simulink model "chap05"  (R2021a)
settings: Solver=FixedStepDiscrete  StartTime=0.0  StopTime=inf  FixedStep=0.001  RelTol=1e-3
undefined symbols (not defined in the file): DiscIntNeverNeededParam, Header, Pose, X, Y, Z
libraries: robotlib x31
(part 1 of 9)
settings Model: Creator=chen  LastModifiedBy=chen
settings OptimizationCC: EnhancedBackFolding=on  PassReuseOutputArgsAs=Individual arguments  ZeroExternalMemoryAtStartup=off  ZeroInternalMemoryAtStartup=off  MaxStackSize=64  OptimizeBlockOrder=speed  DifferentSizesBufferReuse=on  OptimizationCustomize=off  EfficientTunableParamExpr=on
settings DebuggingCC: ParameterTunabilityLossMsg=error
settings HardwareCC: ProdBitPerPointer=32  ProdBitPerSizeT=32  ProdBitPerPtrDiffT=32  ProdLargestAtomicFloat=None  ProdIntDivRoundTo=Undefined  ProdEndianess=Unspecified  ProdWordSize=32  ProdHWDeviceType=Generic->Unspecified (assume 32-bit Generic)
settings SFSimCC: MATLABDynamicMemAlloc=off
settings RTWCC: SystemTargetFile=ert.tlc  HardwareBoard=Robot Operating System (ROS)  TLCOptions="-aInlineSetEventsForThisBaseRateFcn=TLC_FALSE -aSuppressMultiTaskScheduler=TLC_FALSE  -aRateBasedStepFcn=0"  TemplateMakefile=ert_default_tmf  GenerateReport=on  Toolchain=Catkin  LaunchReport=on  TargetLang=C++
settings CodeAppCC: ForceParamTrailComments=on  IgnoreCustomStorageClasses=off  OperatorAnnotations=on  SimulinkDataObjDesc=on  SFDataObjDesc=on  InsertBlockDesc=on
settings ERTTargetCC: SupportContinuousTime=on

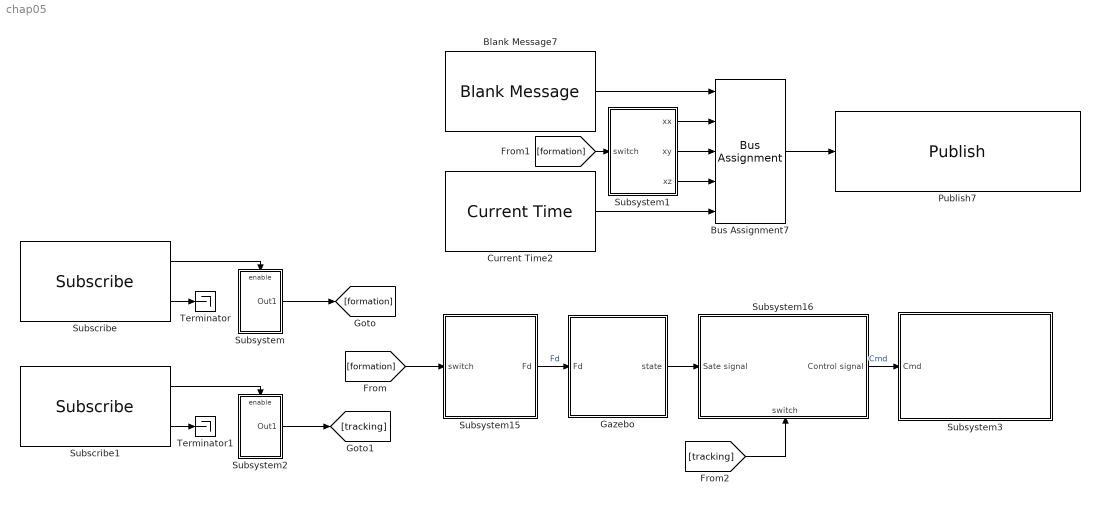
== system chap05 ==
  Blank Message7 : robotlib/Blank Message  messageClass=Message  entityType=geometry_msgs/PoseStamped  messageType=geometry_msgs/PoseStamped  SampleTime=-1  legacyBusStruct=off
  Bus Assignment7 : BusAssignment  AssignedSignals=Pose.Position.X,Pose.Position.Y,Pose.Position.Z,Header.Stamp.Sec
  Current Time2 : robotlib/Current Time  OutputFormat=double  SampleTime=-1  ModelName=chap05
      settings: SourceProductBaseCode=RR
  Gazebo : Subsystem
  Publish7 : robotlib/Publish  topicSource=Specify your own  topic=/uav0/mavros/setpoint_position/local  messageType=geometry_msgs/PoseStamped  legacyBusStruct=off  messageQueueLength=1
  Subscribe : robotlib/Subscribe  topicSource=Specify your own  topic=/start_formation  messageType=std_msgs/Empty  SampleTime=-1  legacyBusStruct=off  messageQueueLength=1
  Subscribe1 : robotlib/Subscribe  topicSource=Specify your own  topic=/start_tracking  messageType=std_msgs/Empty  SampleTime=-1  legacyBusStruct=off  messageQueueLength=1
  Subsystem : Subsystem
  Subsystem1 : Subsystem
  Subsystem15 : Subsystem
  Subsystem16 : Subsystem
      settings: PortSchema="{\"entries\":[{\"content\":{\"sides\":[{\"content\":{\"connectorIds\":[\"In1\"]},\"type\":\"ConnectorPlacement.EquallySpacedRectSide\",\"uuid\":\"50b1559e-7173-4ba8-93e6-314f6d9df527\"},{\"content\":{\"connectorIds\":[\"Out1\"],\"side\":\"RIGHT\"},\"type\":\"ConnectorPlacement.EquallySpacedRectSide\",\"uuid\":\"be527bac-0bcc-4faf-a185-0382edae0189\"},{\"content\":{\"connectorIds\":[],\"side\":\"TOP\"},\"type\":\"ConnectorPlacement.EquallySpacedRectSide\",\"uuid\":\"4c8ef68d-7cf5-4d15-9758-89dbc1169805\"},{\"content\":{\"connectorIds\":[\"In2\"],\"side\":\"BOTTOM\"},\"type\":\"ConnectorPlacement.EquallySpacedRectSide\",\"uuid\":\"887cfce8-f49d-4e35-b980-24c2ad245753\"}]},\"type\":\"ConnectorPlacement.EquallySpacedConnector\",\"uuid\":\"3c2ee67b-c3c9-431a-8107-6d5cd22b236e\"}],\"packageUris\":[\"http://schema.mathworks.com/mf0/Connector/R2020b\"],\"version\":\"1.0\"}"
  Subsystem2 : Subsystem
  Subsystem3 : Subsystem
  Terminator : Terminator
  Terminator1 : Terminator
  wires:
  [formation] -> Subsystem1/1(switch)
  Bus Assignment7/1 -> Publish7/1
  Current Time2/1 -> Bus Assignment7/5
  Blank Message7/1 -> Bus Assignment7/1
  Subsystem16/1(Control signal) -> Subsystem3/1(Cmd)  "Cmd"
  Subsystem1/1(xx) -> Bus Assignment7/2
  Subsystem1/2(xy) -> Bus Assignment7/3
  Subsystem1/3(xz) -> Bus Assignment7/4
  [tracking] -> Subsystem16/2(switch)
  Subscribe/1 -> Subsystem/Enable
  Subscribe/2 -> Terminator/1
  Subscribe1/1 -> Subsystem2/Enable
  Subscribe1/2 -> Terminator1/1
  Subsystem/1(Out1) -> [formation]
  Subsystem2/1(Out1) -> [tracking]
  [formation] -> Subsystem15/1(switch)
  Gazebo/1(state) -> Subsystem16/1(Sate signal)
  Subsystem15/1(Fd) -> Gazebo/1(Fd)  "Fd"

== system chap05/Gazebo ==
  Fd : Inport
  Bus Creator{1..4,6..8} (7 alike) : BusCreator  Inputs=6
  Bus Creator5 : BusCreator  Inputs=7
  Subscribe1 : robotlib/Subscribe  topicSource=Select from ROS network  topic=/uav1/mavros/local_position/velocity_local  messageType=geometry_msgs/TwistStamped  SampleTime=-1  legacyBusStruct=off  messageQueueLength=1
  Subscribe10 : robotlib/Subscribe  topicSource=Select from ROS network  topic=/uav4/mavros/local_position/pose  messageType=geometry_msgs/PoseStamped  SampleTime=-1  legacyBusStruct=off  messageQueueLength=1
  Subscribe11 : robotlib/Subscribe  topicSource=Select from ROS network  topic=/uav5/mavros/local_position/pose  messageType=geometry_msgs/PoseStamped  SampleTime=-1  legacyBusStruct=off  messageQueueLength=1
  Subscribe12 : robotlib/Subscribe  topicSource=Select from ROS network  topic=/uav5/mavros/local_position/velocity_local  messageType=geometry_msgs/TwistStamped  SampleTime=-1  legacyBusStruct=off  messageQueueLength=1
  Subscribe13 : robotlib/Subscribe  topicSource=Select from ROS network  topic=/uav6/mavros/local_position/pose  messageType=geometry_msgs/PoseStamped  SampleTime=-1  legacyBusStruct=off  messageQueueLength=1
  Subscribe14 : robotlib/Subscribe  topicSource=Select from ROS network  topic=/uav6/mavros/local_position/velocity_local  messageType=geometry_msgs/TwistStamped  SampleTime=-1  legacyBusStruct=off  messageQueueLength=1
  Subscribe2 : robotlib/Subscribe  topicSource=Select from ROS network  topic=/uav1/mavros/local_position/pose  messageType=geometry_msgs/PoseStamped  SampleTime=-1  legacyBusStruct=off  messageQueueLength=1
  Subscribe3 : robotlib/Subscribe  topicSource=Select from ROS network  topic=/uav3/mavros/local_position/velocity_local  messageType=geometry_msgs/TwistStamped  SampleTime=-1  legacyBusStruct=off  messageQueueLength=1
  Subscribe4 : robotlib/Subscribe  topicSource=Select from ROS network  topic=/uav3/mavros/local_position/pose  messageType=geometry_msgs/PoseStamped  SampleTime=-1  legacyBusStruct=off  messageQueueLength=1
  Subscribe5 : robotlib/Subscribe  topicSource=Select from ROS network  topic=/uav2/mavros/local_position/velocity_local  messageType=geometry_msgs/TwistStamped  SampleTime=-1  legacyBusStruct=off  messageQueueLength=1
  Subscribe6 : robotlib/Subscribe  topicSource=Select from ROS network  topic=/uav2/mavros/local_position/pose  messageType=geometry_msgs/PoseStamped  SampleTime=-1  legacyBusStruct=off  messageQueueLength=1
  Subscribe7 : robotlib/Subscribe  topicSource=Select from ROS network  topic=/uav0/mavros/local_position/velocity_local  messageType=geometry_msgs/TwistStamped  SampleTime=-1  legacyBusStruct=off  messageQueueLength=1
  Subscribe8 : robotlib/Subscribe  topicSource=Select from ROS network  topic=/uav0/mavros/local_position/pose  messageType=geometry_msgs/PoseStamped  SampleTime=-1  legacyBusStruct=off  messageQueueLength=1
  Subscribe9 : robotlib/Subscribe  topicSource=Select from ROS network  topic=/uav4/mavros/local_position/velocity_local  messageType=geometry_msgs/TwistStamped  SampleTime=-1  legacyBusStruct=off  messageQueueLength=1
  Subsystem1 : Subsystem
  Subsystem2 : Subsystem
  Subsystem3 : Subsystem
  Subsystem4 : Subsystem
  Subsystem5 : Subsystem
  Subsystem6 : Subsystem
  Subsystem7 : Subsystem
  Terminator{,1..6} (7 alike) : Terminator
  state : Outport
  wires:
  Subscribe7/2 -> Subsystem1/2(In2)
  Subscribe8/2 -> Subsystem1/1(In1)
  Subscribe8/1 -> Subsystem1/Enable
  Bus Creator1/1 -> Bus Creator5/1  "node0"
  Subsystem1/6(vz) -> Bus Creator1/6  "vz"
  Subsystem1/5(vy) -> Bus Creator1/5  "vy"
  Subsystem1/1(xx) -> Bus Creator1/1  "xx"
  Subsystem1/2(xy) -> Bus Creator1/2  "xy"
  Subsystem1/4(vx) -> Bus Creator1/4  "vx"
  Subsystem1/3(xz) -> Bus Creator1/3  "xz"
  Subsystem2/3(xz) -> Bus Creator2/3  "xz"
  Subsystem2/4(vx) -> Bus Creator2/4  "vx"
  Subsystem2/2(xy) -> Bus Creator2/2  "xy"
  Subsystem2/1(xx) -> Bus Creator2/1  "xx"
  Subsystem2/5(vy) -> Bus Creator2/5  "vy"
  Subsystem2/6(vz) -> Bus Creator2/6  "vz"
  Bus Creator2/1 -> Bus Creator5/2  "node1"
  Subscribe2/1 -> Subsystem2/Enable
  Subscribe2/2 -> Subsystem2/1(In1)
  Subscribe1/2 -> Subsystem2/2(In2)
  Subscribe1/1 -> Terminator/1
  Subscribe7/1 -> Terminator1/1
  Subscribe5/1 -> Terminator3/1
  Subscribe3/1 -> Terminator2/1
  Subscribe3/2 -> Subsystem4/2(In2)
  Subscribe4/2 -> Subsystem4/1(In1)
  Subscribe4/1 -> Subsystem4/Enable
  Bus Creator4/1 -> Bus Creator5/4  "node3"
  Subsystem4/6(vz) -> Bus Creator4/6  "vz"
  Subsystem4/5(vy) -> Bus Creator4/5  "vy"
  Subsystem4/1(xx) -> Bus Creator4/1  "xx"
  Subsystem4/2(xy) -> Bus Creator4/2  "xy"
  Subsystem4/4(vx) -> Bus Creator4/4  "vx"
  Subsystem4/3(xz) -> Bus Creator4/3  "xz"
  Subsystem3/3(xz) -> Bus Creator3/3  "xz"
  Subsystem3/4(vx) -> Bus Creator3/4  "vx"
  Subsystem3/2(xy) -> Bus Creator3/2  "xy"
  Subsystem3/1(xx) -> Bus Creator3/1  "xx"
  Subsystem3/5(vy) -> Bus Creator3/5  "vy"
  Subsystem3/6(vz) -> Bus Creator3/6  "vz"
  Bus Creator3/1 -> Bus Creator5/3  "node2"
  Subscribe6/1 -> Subsystem3/Enable
  Subscribe6/2 -> Subsystem3/1(In1)
  Subscribe5/2 -> Subsystem3/2(In2)
  Bus Creator5/1 -> state/1
  Subsystem5/3(xz) -> Bus Creator6/3  "xz"
  Subsystem5/4(vx) -> Bus Creator6/4  "vx"
  Subsystem5/2(xy) -> Bus Creator6/2  "xy"
  Subsystem5/1(xx) -> Bus Creator6/1  "xx"
  Subsystem5/5(vy) -> Bus Creator6/5  "vy"
  Subsystem5/6(vz) -> Bus Creator6/6  "vz"
  Bus Creator6/1 -> Bus Creator5/5  "node4"
  Subscribe10/1 -> Subsystem5/Enable
  Subscribe10/2 -> Subsystem5/1(In1)
  Subscribe9/2 -> Subsystem5/2(In2)
  Subscribe9/1 -> Terminator4/1
  Subscribe12/1 -> Terminator5/1
  Subscribe12/2 -> Subsystem6/2(In2)
  Subscribe11/2 -> Subsystem6/1(In1)
  Subscribe11/1 -> Subsystem6/Enable
  Bus Creator7/1 -> Bus Creator5/6  "node5"
  Subsystem6/6(vz) -> Bus Creator7/6  "vz"
  Subsystem6/5(vy) -> Bus Creator7/5  "vy"
  Subsystem6/1(xx) -> Bus Creator7/1  "xx"
  Subsystem6/2(xy) -> Bus Creator7/2  "xy"
  Subsystem6/4(vx) -> Bus Creator7/4  "vx"
  Subsystem6/3(xz) -> Bus Creator7/3  "xz"
  Subsystem7/3(xz) -> Bus Creator8/3  "xz"
  Subsystem7/4(vx) -> Bus Creator8/4  "vx"
  Subsystem7/2(xy) -> Bus Creator8/2  "xy"
  Subsystem7/1(xx) -> Bus Creator8/1  "xx"
  Subsystem7/5(vy) -> Bus Creator8/5  "vy"
  Subsystem7/6(vz) -> Bus Creator8/6  "vz"
  Bus Creator8/1 -> Bus Creator5/7  "node6"
  Subscribe13/1 -> Subsystem7/Enable
  Subscribe13/2 -> Subsystem7/1(In1)
  Subscribe14/2 -> Subsystem7/2(In2)
  Subscribe14/1 -> Terminator6/1
  Fd/1 -> Subsystem2/3(Fd), Subsystem4/3(Fd), Subsystem7/3(Fd), Subsystem6/3(Fd), Subsystem5/3(Fd), Subsystem3/3(Fd)

== system chap05/Subsystem ==
  Enable : EnablePort
  Constant3 : Constant
  Out1 : Outport  InitialOutput=0
  wires:
  Constant3/1 -> Out1/1

== system chap05/Subsystem1 ==
  switch : Inport
  Add{1..4} (4 alike) : Sum
  Constant : Constant  Value=2.5
  Constant1 : Constant  Value=pi
  Constant3 : Constant  Value=0.214
  Constant4 : Constant  Value=0.35
  Constant5 : Constant  Value=0
  Constant6 : Constant  Value=0.214
  Constant8 : Constant  Value=0.5*pi
  Product{,1..3,5} (5 alike) : Product
  Subsystem : Subsystem
      settings: PortSchema="{\"entries\":[{\"content\":{\"sides\":[{\"content\":{\"connectorIds\":[\"In1\"]},\"type\":\"ConnectorPlacement.EquallySpacedRectSide\",\"uuid\":\"50b1559e-7173-4ba8-93e6-314f6d9df527\"},{\"content\":{\"connectorIds\":[\"Out1\"],\"side\":\"RIGHT\"},\"type\":\"ConnectorPlacement.EquallySpacedRectSide\",\"uuid\":\"be527bac-0bcc-4faf-a185-0382edae0189\"},{\"content\":{\"connectorIds\":[\"In2\"],\"side\":\"TOP\"},\"type\":\"ConnectorPlacement.EquallySpacedRectSide\",\"uuid\":\"4c8ef68d-7cf5-4d15-9758-89dbc1169805\"}]},\"type\":\"ConnectorPlacement.EquallySpacedConnector\",\"uuid\":\"3c2ee67b-c3c9-431a-8107-6d5cd22b236e\"}],\"packageUris\":[\"http://schema.mathworks.com/mf0/Connector/R2020b\"],\"version\":\"1.0\"}"
  Subsystem1 : Subsystem
      settings: PortSchema="{\"entries\":[{\"content\":{\"sides\":[{\"content\":{\"connectorIds\":[\"In1\"]},\"type\":\"ConnectorPlacement.EquallySpacedRectSide\",\"uuid\":\"50b1559e-7173-4ba8-93e6-314f6d9df527\"},{\"content\":{\"connectorIds\":[\"Out1\"],\"side\":\"RIGHT\"},\"type\":\"ConnectorPlacement.EquallySpacedRectSide\",\"uuid\":\"be527bac-0bcc-4faf-a185-0382edae0189\"},{\"content\":{\"connectorIds\":[\"In2\"],\"side\":\"TOP\"},\"type\":\"ConnectorPlacement.EquallySpacedRectSide\",\"uuid\":\"4c8ef68d-7cf5-4d15-9758-89dbc1169805\"}]},\"type\":\"ConnectorPlacement.EquallySpacedConnector\",\"uuid\":\"3c2ee67b-c3c9-431a-8107-6d5cd22b236e\"}],\"packageUris\":[\"http://schema.mathworks.com/mf0/Connector/R2020b\"],\"version\":\"1.0\"}"
  Subsystem16 : Subsystem
  Trigonometric Function : Trigonometry  Operator=cos
  Trigonometric Function2 : Trigonometry  Operator=cos
  r1 : Constant  Value=4
  r2 : Constant  Value=1.5
  xx : Outport
  xy : Outport  Port=2
  xz : Outport  Port=3
  wires:
  Add2/1 -> Trigonometric Function2/1
  Trigonometric Function2/1 -> Product2/2
  Product2/1 -> Subsystem1/1(zt3)
  r1/1 -> Product2/1
  [time] -> Product5/2
  Product5/1 -> Add1/1
  Constant4/1 -> Product5/1
  Constant5/1 -> Add1/2
  Constant8/1 -> Add2/2
  Constant6/1 -> Product3/1
  [time] -> Product3/2
  Product3/1 -> Add2/1
  Trigonometric Function/1 -> Product/2
  r2/1 -> Product/1
  Add3/1 -> Trigonometric Function/1
  [time] -> Product1/2
  Constant3/1 -> Product1/1
  Product/1 -> Add4/1
  Constant/1 -> Add4/2
  Product1/1 -> Add3/1
  Constant1/1 -> Add3/2
  Add4/1 -> Subsystem/1(zt3)
  Subsystem16/1(time) -> [time]
  switch/1 -> [switch], Subsystem16/1(switch)
  Subsystem/1(Out1) -> xz/1
  [switch] -> Subsystem/2(switch)
  Subsystem1/1(xy) -> xy/1
  [switch] -> Subsystem1/2(switch)
  Add1/1 -> xx/1

== system chap05/Subsystem15 ==
  switch : Inport
  Subsystem : Subsystem
  Subsystem14 : Subsystem
  Subsystem16 : Subsystem
  Subsystem8 : Subsystem
  Switch : Switch  Criteria=u2 > Threshold  Threshold=10
  Switch1 : Switch  Criteria=u2 > Threshold  Threshold=20
  Fd : Outport
  wires:
  Switch/1 -> Switch1/3
  Subsystem16/1(time) -> Switch/2, Switch1/2
  switch/1 -> Subsystem16/1(switch)
  Subsystem14/1(Fd3) -> Switch1/1
  Subsystem8/1(Fd1) -> Switch/3
  Subsystem/1(Fd2) -> Switch/1
  Switch1/1 -> Fd/1

== system chap05/Subsystem16 ==
  Sate signal : Inport
  switch : Inport  Port=2
  Bus Creator : BusCreator  Inputs=6
  Bus Creator2 : BusCreator  Inputs=3
  Bus Creator3 : BusCreator  Inputs=6
  Subsystem : Subsystem
      settings: PortSchema="{\"entries\":[{\"content\":{\"sides\":[{\"content\":{\"connectorIds\":[\"In1\"]},\"type\":\"ConnectorPlacement.EquallySpacedRectSide\",\"uuid\":\"50b1559e-7173-4ba8-93e6-314f6d9df527\"},{\"content\":{\"connectorIds\":[\"Out1\"],\"side\":\"RIGHT\"},\"type\":\"ConnectorPlacement.EquallySpacedRectSide\",\"uuid\":\"be527bac-0bcc-4faf-a185-0382edae0189\"},{\"content\":{\"connectorIds\":[],\"side\":\"TOP\"},\"type\":\"ConnectorPlacement.EquallySpacedRectSide\",\"uuid\":\"4c8ef68d-7cf5-4d15-9758-89dbc1169805\"},{\"content\":{\"connectorIds\":[\"In2\"],\"side\":\"BOTTOM\"},\"type\":\"ConnectorPlacement.EquallySpacedRectSide\",\"uuid\":\"2cbbf04f-3669-4691-b0be-f4c904003730\"}]},\"type\":\"ConnectorPlacement.EquallySpacedConnector\",\"uuid\":\"3c2ee67b-c3c9-431a-8107-6d5cd22b236e\"}],\"packageUris\":[\"http://schema.mathworks.com/mf0/Connector/R2020b\"],\"version\":\"1.0\"}"
  Subsystem1 : Subsystem
      settings: PortSchema="{\"entries\":[{\"content\":{\"sides\":[{\"content\":{\"connectorIds\":[\"In1\"]},\"type\":\"ConnectorPlacement.EquallySpacedRectSide\",\"uuid\":\"50b1559e-7173-4ba8-93e6-314f6d9df527\"},{\"content\":{\"connectorIds\":[\"Out1\"],\"side\":\"RIGHT\"},\"type\":\"ConnectorPlacement.EquallySpacedRectSide\",\"uuid\":\"be527bac-0bcc-4faf-a185-0382edae0189\"},{\"content\":{\"connectorIds\":[],\"side\":\"TOP\"},\"type\":\"ConnectorPlacement.EquallySpacedRectSide\",\"uuid\":\"4c8ef68d-7cf5-4d15-9758-89dbc1169805\"},{\"content\":{\"connectorIds\":[\"In2\"],\"side\":\"BOTTOM\"},\"type\":\"ConnectorPlacement.EquallySpacedRectSide\",\"uuid\":\"62a0e2ad-d0ed-4a01-9855-22721dd4145c\"}]},\"type\":\"ConnectorPlacement.EquallySpacedConnector\",\"uuid\":\"3c2ee67b-c3c9-431a-8107-6d5cd22b236e\"}],\"packageUris\":[\"http://schema.mathworks.com/mf0/Connector/R2020b\"],\"version\":\"1.0\"}"
  Subsystem12 : Subsystem
  Subsystem14 : Subsystem
  Subsystem15 : Subsystem
  Subsystem16 : Subsystem
  Subsystem17 : Subsystem
  Subsystem2 : Subsystem
      settings: PortSchema="{\"entries\":[{\"content\":{\"sides\":[{\"content\":{\"connectorIds\":[\"In1\"]},\"type\":\"ConnectorPlacement.EquallySpacedRectSide\",\"uuid\":\"50b1559e-7173-4ba8-93e6-314f6d9df527\"},{\"content\":{\"connectorIds\":[\"Out1\"],\"side\":\"RIGHT\"},\"type\":\"ConnectorPlacement.EquallySpacedRectSide\",\"uuid\":\"be527bac-0bcc-4faf-a185-0382edae0189\"},{\"content\":{\"connectorIds\":[],\"side\":\"TOP\"},\"type\":\"ConnectorPlacement.EquallySpacedRectSide\",\"uuid\":\"4c8ef68d-7cf5-4d15-9758-89dbc1169805\"},{\"content\":{\"connectorIds\":[\"In2\"],\"side\":\"BOTTOM\"},\"type\":\"ConnectorPlacement.EquallySpacedRectSide\",\"uuid\":\"45420c28-548a-43d1-89f9-1bbe4c81c7d8\"}]},\"type\":\"ConnectorPlacement.EquallySpacedConnector\",\"uuid\":\"3c2ee67b-c3c9-431a-8107-6d5cd22b236e\"}],\"packageUris\":[\"http://schema.mathworks.com/mf0/Connector/R2020b\"],\"version\":\"1.0\"}"
  Subsystem3 : Subsystem
      settings: PortSchema="{\"entries\":[{\"content\":{\"sides\":[{\"content\":{\"connectorIds\":[\"In1\"]},\"type\":\"ConnectorPlacement.EquallySpacedRectSide\",\"uuid\":\"50b1559e-7173-4ba8-93e6-314f6d9df527\"},{\"content\":{\"connectorIds\":[\"Out1\"],\"side\":\"RIGHT\"},\"type\":\"ConnectorPlacement.EquallySpacedRectSide\",\"uuid\":\"be527bac-0bcc-4faf-a185-0382edae0189\"},{\"content\":{\"connectorIds\":[],\"side\":\"TOP\"},\"type\":\"ConnectorPlacement.EquallySpacedRectSide\",\"uuid\":\"4c8ef68d-7cf5-4d15-9758-89dbc1169805\"},{\"content\":{\"connectorIds\":[\"In2\"],\"side\":\"BOTTOM\"},\"type\":\"ConnectorPlacement.EquallySpacedRectSide\",\"uuid\":\"05de88b9-9e0a-48cf-94d1-e5072cafba72\"}]},\"type\":\"ConnectorPlacement.EquallySpacedConnector\",\"uuid\":\"3c2ee67b-c3c9-431a-8107-6d5cd22b236e\"}],\"packageUris\":[\"http://schema.mathworks.com/mf0/Connector/R2020b\"],\"version\":\"1.0\"}"
  Subsystem5 : Subsystem
      settings: PortSchema="{\"entries\":[{\"content\":{\"sides\":[{\"content\":{\"connectorIds\":[\"In1\"]},\"type\":\"ConnectorPlacement.EquallySpacedRectSide\",\"uuid\":\"50b1559e-7173-4ba8-93e6-314f6d9df527\"},{\"content\":{\"connectorIds\":[\"Out1\"],\"side\":\"RIGHT\"},\"type\":\"ConnectorPlacement.EquallySpacedRectSide\",\"uuid\":\"be527bac-0bcc-4faf-a185-0382edae0189\"},{\"content\":{\"connectorIds\":[],\"side\":\"TOP\"},\"type\":\"ConnectorPlacement.EquallySpacedRectSide\",\"uuid\":\"4c8ef68d-7cf5-4d15-9758-89dbc1169805\"},{\"content\":{\"connectorIds\":[\"In2\"],\"side\":\"BOTTOM\"},\"type\":\"ConnectorPlacement.EquallySpacedRectSide\",\"uuid\":\"45d8b813-fb3b-4390-971a-06d0d1d89687\"}]},\"type\":\"ConnectorPlacement.EquallySpacedConnector\",\"uuid\":\"3c2ee67b-c3c9-431a-8107-6d5cd22b236e\"}],\"packageUris\":[\"http://schema.mathworks.com/mf0/Connector/R2020b\"],\"version\":\"1.0\"}"
  Subsystem6 : Subsystem
      settings: PortSchema="{\"entries\":[{\"content\":{\"sides\":[{\"content\":{\"connectorIds\":[\"In1\"]},\"type\":\"ConnectorPlacement.EquallySpacedRectSide\",\"uuid\":\"50b1559e-7173-4ba8-93e6-314f6d9df527\"},{\"content\":{\"connectorIds\":[\"Out1\"],\"side\":\"RIGHT\"},\"type\":\"ConnectorPlacement.EquallySpacedRectSide\",\"uuid\":\"be527bac-0bcc-4faf-a185-0382edae0189\"},{\"content\":{\"connectorIds\":[],\"side\":\"TOP\"},\"type\":\"ConnectorPlacement.EquallySpacedRectSide\",\"uuid\":\"4c8ef68d-7cf5-4d15-9758-89dbc1169805\"},{\"content\":{\"connectorIds\":[\"In2\"],\"side\":\"BOTTOM\"},\"type\":\"ConnectorPlacement.EquallySpacedRectSide\",\"uuid\":\"7372fe2b-1118-4856-9e0f-b588141a0ffd\"}]},\"type\":\"ConnectorPlacement.EquallySpacedConnector\",\"uuid\":\"3c2ee67b-c3c9-431a-8107-6d5cd22b236e\"}],\"packageUris\":[\"http://schema.mathworks.com/mf0/Connector/R2020b\"],\"version\":\"1.0\"}"
  Subsystem8 : Subsystem
  Control signal : Outport
  wires:
  Subsystem5/1(u3) -> Bus Creator/3
  Subsystem3/1(u4) -> Bus Creator/4
  Subsystem1/1(u5) -> Bus Creator/5
  Subsystem/1(u1) -> Bus Creator/1
  Subsystem2/1(u2) -> Bus Creator/2
  Bus Creator/1 -> [control], Control signal/1
  Sate signal/1 -> Bus Creator2/2  "state(t)"
  [control] -> Bus Creator2/3  "control"
  Subsystem15/1(u2) -> Bus Creator3/2
  Subsystem8/1(u4) -> Bus Creator3/4
  Subsystem12/1(u6) -> Bus Creator3/6
  Subsystem16/1(u5) -> Bus Creator3/5
  Subsystem14/1(u1) -> Bus Creator3/1
  Bus Creator3/1 -> Bus Creator2/1  "state(tk)"
  Subsystem17/1(u3) -> Bus Creator3/3
  Subsystem6/1(u6) -> Bus Creator/6
  switch/1 -> Subsystem6/2(switch), Subsystem1/2(switch), Subsystem3/2(switch), Subsystem5/2(switch), Subsystem2/2(switch), Subsystem/2(switch)
  Bus Creator2/1 -> Subsystem3/1(In19), Subsystem1/1(In19), Subsystem6/1(In19), Subsystem15/1(In19), Subsystem17/1(In19), Subsystem16/1(In19), Subsystem12/1(In19), Subsystem8/1(In19), Subsystem14/1(In19), Subsystem/1(In19), Subsystem2/1(In19), Subsystem5/1(In19)

== system chap05/Subsystem2 ==
  Enable : EnablePort
  Constant3 : Constant  Value=0
  Out1 : Outport  InitialOutput=0
  wires:
  Constant3/1 -> Out1/1

== system chap05/Subsystem3 ==
  Cmd : Inport
  Blank Message{1..6} (6 alike) : robotlib/Blank Message  messageClass=Message  entityType=geometry_msgs/Vector3  messageType=geometry_msgs/Vector3  SampleTime=-1  legacyBusStruct=off
  Bus Assignment{1..6} (6 alike) : BusAssignment  AssignedSignals=X,Y,Z
  Bus Selector : BusSelector  OutputSignals=node1.ux,node1.uy,node1.uz
  Bus Selector1 : BusSelector  OutputSignals=node3.ux,node3.uy,node3.uz
  Bus Selector2 : BusSelector  OutputSignals=node4.ux,node4.uy,node4.uz
  Bus Selector3 : BusSelector  OutputSignals=node5.ux,node5.uy,node5.uz
  Bus Selector4 : BusSelector  OutputSignals=node6.ux,node6.uy,node6.uz
  Bus Selector7 : BusSelector  OutputSignals=node2.ux,node2.uy,node2.uz
  Publish1 : robotlib/Publish  topicSource=Specify your own  topic=/uav2/accel_control  messageType=geometry_msgs/Vector3  legacyBusStruct=off  messageQueueLength=1
  Publish2 : robotlib/Publish  topicSource=Specify your own  topic=/uav1/accel_control  messageType=geometry_msgs/Vector3  legacyBusStruct=off  messageQueueLength=1
  Publish3 : robotlib/Publish  topicSource=Specify your own  topic=/uav3/accel_control  messageType=geometry_msgs/Vector3  legacyBusStruct=off  messageQueueLength=1
  Publish4 : robotlib/Publish  topicSource=Specify your own  topic=/uav4/accel_control  messageType=geometry_msgs/Vector3  legacyBusStruct=off  messageQueueLength=1
  Publish5 : robotlib/Publish  topicSource=Specify your own  topic=/uav5/accel_control  messageType=geometry_msgs/Vector3  legacyBusStruct=off  messageQueueLength=1
  Publish6 : robotlib/Publish  topicSource=Specify your own  topic=/uav6/accel_control  messageType=geometry_msgs/Vector3  legacyBusStruct=off  messageQueueLength=1
  wires:
  Bus Selector/1 -> Bus Assignment2/2  "<ux>"
  Blank Message1/1 -> Bus Assignment2/1
  Bus Selector/3 -> Bus Assignment2/4  "<uz>"
  Bus Selector7/2 -> Bus Assignment1/3  "<uy>"
  Bus Selector7/1 -> Bus Assignment1/2  "<ux>"
  Blank Message2/1 -> Bus Assignment1/1
  Bus Assignment2/1 -> Publish2/1
  Bus Selector7/3 -> Bus Assignment1/4  "<uz>"
  Bus Assignment1/1 -> Publish1/1
  Bus Selector/2 -> Bus Assignment2/3  "<uy>"
  Bus Assignment3/1 -> Publish3/1
  Bus Selector1/3 -> Bus Assignment3/4  "<uz>"
  Blank Message3/1 -> Bus Assignment3/1
  Bus Selector1/1 -> Bus Assignment3/2  "<ux>"
  Bus Selector1/2 -> Bus Assignment3/3  "<uy>"
  Bus Selector2/2 -> Bus Assignment4/3  "<uy>"
  Bus Selector2/1 -> Bus Assignment4/2  "<ux>"
  Blank Message4/1 -> Bus Assignment4/1
  Bus Selector2/3 -> Bus Assignment4/4  "<uz>"
  Bus Assignment4/1 -> Publish4/1
  Bus Assignment5/1 -> Publish5/1
  Bus Selector3/3 -> Bus Assignment5/4  "<uz>"
  Blank Message5/1 -> Bus Assignment5/1
  Bus Selector3/1 -> Bus Assignment5/2  "<ux>"
  Bus Selector3/2 -> Bus Assignment5/3  "<uy>"
  Bus Selector4/2 -> Bus Assignment6/3  "<uy>"
  Bus Selector4/1 -> Bus Assignment6/2  "<ux>"
  Blank Message6/1 -> Bus Assignment6/1
  Bus Selector4/3 -> Bus Assignment6/4  "<uz>"
  Bus Assignment6/1 -> Publish6/1
  Cmd/1 -> Bus Selector/1, Bus Selector7/1, Bus Selector1/1, Bus Selector2/1, Bus Selector4/1, Bus Selector3/1

== system chap05/Gazebo/Subsystem1 ==
  In1 : Inport
  In2 : Inport  Port=2
  Enable : EnablePort
  Bus Selector1 : BusSelector  OutputSignals=Twist.Linear.X,Twist.Linear.Y,Twist.Linear.Z
  Bus Selector4 : BusSelector  OutputSignals=Pose.Position.X,Pose.Position.Y,Pose.Position.Z
  Subsystem3 : Subsystem
  xx : Outport
  xy : Outport  Port=2
  xz : Outport  Port=3
  vx : Outport  Port=4
  vy : Outport  Port=5
  vz : Outport  Port=6
  wires:
  Bus Selector1/3 -> vz/1  "<Z>"
  In2/1 -> Bus Selector1/1
  Bus Selector1/1 -> vx/1  "<X>"
  Bus Selector1/2 -> vy/1  "<Y>"
  Bus Selector4/1 -> Subsystem3/1(In1)  "<X>"
  In1/1 -> Bus Selector4/1
  Bus Selector4/2 -> xy/1  "<Y>"
  Bus Selector4/3 -> xz/1  "<Z>"
  Subsystem3/1(Out1) -> xx/1

== system chap05/Gazebo/Subsystem2 ==
  In1 : Inport
  In2 : Inport  Port=2
  Fd : Inport  Port=3
  Enable : EnablePort
  Add3 : Sum  Inputs=-+
  Add4 : Sum  Inputs=-+
  Add5 : Sum  Inputs=-+
  Bus Selector1 : BusSelector  OutputSignals=Twist.Linear.X,Twist.Linear.Y,Twist.Linear.Z
  Bus Selector2 : BusSelector  OutputSignals=pd1.xx,pd1.xy,pd1.xz
  Bus Selector4 : BusSelector  OutputSignals=Pose.Position.X,Pose.Position.Y,Pose.Position.Z
  Subsystem3 : Subsystem
  Subsystem4 : Subsystem
  xx : Outport
  xy : Outport  Port=2
  xz : Outport  Port=3
  vx : Outport  Port=4
  vy : Outport  Port=5
  vz : Outport  Port=6
  wires:
  In1/1 -> Bus Selector4/1
  Bus Selector4/1 -> Subsystem3/1(In1)  "<X>"
  Bus Selector4/2 -> Subsystem4/1(In1)  "<Y>"
  Bus Selector1/2 -> vy/1  "<Y>"
  Bus Selector1/1 -> vx/1  "<X>"
  In2/1 -> Bus Selector1/1
  Bus Selector1/3 -> vz/1  "<Z>"
  Add5/1 -> xz/1
  Add4/1 -> xy/1
  Add3/1 -> xx/1
  Subsystem4/1(Out1) -> Add4/2
  Bus Selector4/3 -> Add5/2  "<Z>"
  Bus Selector2/2 -> Add4/1  "<xy>"
  Fd/1 -> Bus Selector2/1
  Bus Selector2/1 -> Add3/1  "<xx>"
  Subsystem3/1(Out1) -> Add3/2
  Bus Selector2/3 -> Add5/1  "<xz>"

== system chap05/Gazebo/Subsystem3 ==
  In1 : Inport
  In2 : Inport  Port=2
  Fd : Inport  Port=3
  Enable : EnablePort
  Add3 : Sum  Inputs=-+
  Add4 : Sum  Inputs=-+
  Add5 : Sum  Inputs=-+
  Bus Selector1 : BusSelector  OutputSignals=Twist.Linear.X,Twist.Linear.Y,Twist.Linear.Z
  Bus Selector2 : BusSelector  OutputSignals=pd2.xx,pd2.xy,pd2.xz
  Bus Selector4 : BusSelector  OutputSignals=Pose.Position.X,Pose.Position.Y,Pose.Position.Z
  Subsystem3 : Subsystem
  Subsystem4 : Subsystem
  xx : Outport
  xy : Outport  Port=2
  xz : Outport  Port=3
  vx : Outport  Port=4
  vy : Outport  Port=5
  vz : Outport  Port=6
  wires:
  Subsystem4/1(Out1) -> Add4/2
  Bus Selector1/3 -> vz/1  "<Z>"
  In2/1 -> Bus Selector1/1
  Bus Selector1/1 -> vx/1  "<X>"
  Bus Selector1/2 -> vy/1  "<Y>"
  Bus Selector4/2 -> Subsystem4/1(In1)  "<Y>"
  Bus Selector4/1 -> Subsystem3/1(In1)  "<X>"
  In1/1 -> Bus Selector4/1
  Bus Selector4/3 -> Add5/2  "<Z>"
  Bus Selector2/1 -> Add3/1  "<xx>"
  Bus Selector2/2 -> Add4/1  "<xy>"
  Bus Selector2/3 -> Add5/1  "<xz>"
  Fd/1 -> Bus Selector2/1
  Subsystem3/1(Out1) -> Add3/2
  Add3/1 -> xx/1
  Add4/1 -> xy/1
  Add5/1 -> xz/1

== system chap05/Gazebo/Subsystem4 ==
  In1 : Inport
  In2 : Inport  Port=2
  Fd : Inport  Port=3
  Enable : EnablePort
  Add3 : Sum  Inputs=-+
  Add4 : Sum  Inputs=-+
  Add5 : Sum  Inputs=-+
  Bus Selector1 : BusSelector  OutputSignals=Twist.Linear.X,Twist.Linear.Y,Twist.Linear.Z
  Bus Selector2 : BusSelector  OutputSignals=pd3.xx,pd3.xy,pd3.xz
  Bus Selector4 : BusSelector  OutputSignals=Pose.Position.X,Pose.Position.Y,Pose.Position.Z
  Subsystem1 : Subsystem
  Subsystem2 : Subsystem
  xx : Outport
  xy : Outport  Port=2
  xz : Outport  Port=3
  vx : Outport  Port=4
  vy : Outport  Port=5
  vz : Outport  Port=6
  wires:
  Fd/1 -> Bus Selector2/1
  Bus Selector2/3 -> Add5/1  "<xz>"
  Bus Selector2/2 -> Add4/1  "<xy>"
  Bus Selector2/1 -> Add3/1  "<xx>"
  Add3/1 -> xx/1  "xx"
  Add5/1 -> xz/1  "xz"
  Add4/1 -> xy/1  "xy"
  Bus Selector4/3 -> Add5/2  "<Z>"
  In1/1 -> Bus Selector4/1
  Bus Selector4/1 -> Subsystem1/1(In1)  "<X>"
  Bus Selector4/2 -> Subsystem2/1(In1)  "<Y>"
  Bus Selector1/2 -> vy/1  "<Y>"
  Bus Selector1/1 -> vx/1  "<X>"
  In2/1 -> Bus Selector1/1
  Bus Selector1/3 -> vz/1  "<Z>"
  Subsystem2/1(Out1) -> Add4/2
  Subsystem1/1(Out1) -> Add3/2

== system chap05/Gazebo/Subsystem5 ==
  In1 : Inport
  In2 : Inport  Port=2
  Fd : Inport  Port=3
  Enable : EnablePort
  Add3 : Sum  Inputs=-+
  Add4 : Sum  Inputs=-+
  Add5 : Sum  Inputs=-+
  Bus Selector1 : BusSelector  OutputSignals=Twist.Linear.X,Twist.Linear.Y,Twist.Linear.Z
  Bus Selector2 : BusSelector  OutputSignals=pd4.xx,pd4.xy,pd4.xz
  Bus Selector4 : BusSelector  OutputSignals=Pose.Position.X,Pose.Position.Y,Pose.Position.Z
  Subsystem1 : Subsystem
  Subsystem2 : Subsystem
  xx : Outport
  xy : Outport  Port=2
  xz : Outport  Port=3
  vx : Outport  Port=4
  vy : Outport  Port=5
  vz : Outport  Port=6
  wires:
  Subsystem2/1(Out1) -> Add4/2
  Bus Selector1/3 -> vz/1  "<Z>"
  In2/1 -> Bus Selector1/1
  Bus Selector1/1 -> vx/1  "<X>"
  Bus Selector1/2 -> vy/1  "<Y>"
  Bus Selector4/2 -> Subsystem2/1(In1)  "<Y>"
  Bus Selector4/1 -> Subsystem1/1(In1)  "<X>"
  In1/1 -> Bus Selector4/1
  Bus Selector4/3 -> Add5/2  "<Z>"
  Add4/1 -> xy/1  "xy"
  Add5/1 -> xz/1  "xz"
  Add3/1 -> xx/1  "xx"
  Bus Selector2/1 -> Add3/1  "<xx>"
  Bus Selector2/2 -> Add4/1  "<xy>"
  Bus Selector2/3 -> Add5/1  "<xz>"
  Fd/1 -> Bus Selector2/1
  Subsystem1/1(Out1) -> Add3/2

== system chap05/Gazebo/Subsystem6 ==
  In1 : Inport
  In2 : Inport  Port=2
  Fd : Inport  Port=3
  Enable : EnablePort
  Add3 : Sum  Inputs=-+
  Add4 : Sum  Inputs=-+
  Add5 : Sum  Inputs=-+
  Bus Selector1 : BusSelector  OutputSignals=Twist.Linear.X,Twist.Linear.Y,Twist.Linear.Z
  Bus Selector2 : BusSelector  OutputSignals=pd5.xx,pd5.xy,pd5.xz
  Bus Selector4 : BusSelector  OutputSignals=Pose.Position.X,Pose.Position.Y,Pose.Position.Z
  Subsystem1 : Subsystem
  Subsystem2 : Subsystem
  xx : Outport
  xy : Outport  Port=2
  xz : Outport  Port=3
  vx : Outport  Port=4
  vy : Outport  Port=5
  vz : Outport  Port=6
  wires:
  Fd/1 -> Bus Selector2/1
  Bus Selector2/3 -> Add5/1  "<xz>"
  Bus Selector2/2 -> Add4/1  "<xy>"
  Bus Selector2/1 -> Add3/1  "<xx>"
  Add3/1 -> xx/1  "xx"
  Add5/1 -> xz/1  "xz"
  Add4/1 -> xy/1  "xy"
  Bus Selector4/3 -> Add5/2  "<Z>"
  In1/1 -> Bus Selector4/1
  Bus Selector4/1 -> Subsystem1/1(In1)  "<X>"
  Bus Selector4/2 -> Subsystem2/1(In1)  "<Y>"
  Bus Selector1/2 -> vy/1  "<Y>"
  Bus Selector1/1 -> vx/1  "<X>"
  In2/1 -> Bus Selector1/1
  Bus Selector1/3 -> vz/1  "<Z>"
  Subsystem2/1(Out1) -> Add4/2
  Subsystem1/1(Out1) -> Add3/2

== system chap05/Gazebo/Subsystem7 ==
  In1 : Inport
  In2 : Inport  Port=2
  Fd : Inport  Port=3
  Enable : EnablePort
  Add3 : Sum  Inputs=-+
  Add4 : Sum  Inputs=-+
  Add5 : Sum  Inputs=-+
  Bus Selector1 : BusSelector  OutputSignals=Twist.Linear.X,Twist.Linear.Y,Twist.Linear.Z
  Bus Selector2 : BusSelector  OutputSignals=pd6.xx,pd6.xy,pd6.xz
  Bus Selector4 : BusSelector  OutputSignals=Pose.Position.X,Pose.Position.Y,Pose.Position.Z
  Subsystem1 : Subsystem
  Subsystem2 : Subsystem
  xx : Outport
  xy : Outport  Port=2
  xz : Outport  Port=3
  vx : Outport  Port=4
  vy : Outport  Port=5
  vz : Outport  Port=6
  wires:
  Subsystem2/1(Out1) -> Add4/2
  Bus Selector1/3 -> vz/1  "<Z>"
  In2/1 -> Bus Selector1/1
  Bus Selector1/1 -> vx/1  "<X>"
  Bus Selector1/2 -> vy/1  "<Y>"
  Bus Selector4/2 -> Subsystem2/1(In1)  "<Y>"
  Bus Selector4/1 -> Subsystem1/1(In1)  "<X>"
  In1/1 -> Bus Selector4/1
  Bus Selector4/3 -> Add5/2  "<Z>"
  Add4/1 -> xy/1  "xy"
  Add5/1 -> xz/1  "xz"
  Add3/1 -> xx/1  "xx"
  Bus Selector2/1 -> Add3/1  "<xx>"
  Bus Selector2/2 -> Add4/1  "<xy>"
  Bus Selector2/3 -> Add5/1  "<xz>"
  Fd/1 -> Bus Selector2/1
  Subsystem1/1(Out1) -> Add3/2

== system chap05/Subsystem1/Subsystem ==
  zt3 : Inport
  switch : Inport  Port=2
  Constant4 : Constant
  Switch1 : Switch  Criteria=u2 > Threshold
  Out1 : Outport
  wires:
  Constant4/1 -> Switch1/3
  switch/1 -> Switch1/2
  Switch1/1 -> Out1/1
  zt3/1 -> Switch1/1

== system chap05/Subsystem1/Subsystem1 ==
  zt3 : Inport
  switch : Inport  Port=2
  Constant4 : Constant  Value=0
  Switch1 : Switch  Criteria=u2 > Threshold
  xy : Outport
  wires:
  zt3/1 -> Switch1/1
  Switch1/1 -> xy/1
  switch/1 -> Switch1/2
  Constant4/1 -> Switch1/3

== system chap05/Subsystem1/Subsystem16 ==
  switch : Inport
  Add : Sum
  Constant1 : Constant  Value=0
  Data Store Memory : DataStoreMemory  ReadBeforeWriteMsg=warning  WriteAfterWriteMsg=warning  WriteAfterReadMsg=warning  ShowAdditionalParam=off
  Data Store Read : DataStoreRead  IndexOptions=Index vector (dialog)  Indices=1  OutputSizes=1
  Data Store Write : DataStoreWrite  IndexOptions=Index vector (dialog)  Indices=1  OutputSizes=1
  Switch : Switch  Criteria=u2 > Threshold
  t : Constant  Value=0.001
  time : Outport
  wires:
  Constant1/1 -> Switch/3
  Add/1 -> Data Store Write/1
  Switch/1 -> Add/1
  t/1 -> Switch/1
  switch/1 -> Switch/2
  Data Store Read/1 -> time/1, Add/2

== system chap05/Subsystem15/Subsystem ==
  note: f1 = [-1  1 0];
      |  f2 = [ 0  1 0];
      |  f3 = [ 1  1 0];
      |  f4 = [-1 -1 0];
      |  f5 = [ 0 -1 0];
      |  f6 = [ 1 -1 0];
  note: % fx2 = [-1 1 0
      | % 1 1 0
      | % 2 0 0
      | % -2 0 0
      | % -1 -1 0
      | % 1 -1 0];
  Bus Creator{,2..6} (6 alike) : BusCreator  Inputs=3
  Bus Creator1 : BusCreator  Inputs=6
  Constant{,12,14..15} (4 alike) : Constant  Value=-1
  Constant{1,3..4,17} (4 alike) : Constant
  Constant{2,5,7..8,10..11,13,16} (8 alike) : Constant  Value=0
  Constant6 : Constant  Value=2
  Constant9 : Constant  Value=-2
  Fd2 : Outport
  wires:
  Constant/1 -> Bus Creator/1  "xx"
  Bus Creator/1 -> Bus Creator1/1  "pd1"
  Constant2/1 -> Bus Creator/3  "xz"
  Constant1/1 -> Bus Creator/2  "xy"
  Constant4/1 -> Bus Creator2/2  "xy"
  Constant5/1 -> Bus Creator2/3  "xz"
  Bus Creator2/1 -> Bus Creator1/2  "pd2"
  Constant3/1 -> Bus Creator2/1  "xx"
  Bus Creator3/1 -> Bus Creator1/3  "pd3"
  Bus Creator6/1 -> Bus Creator1/6  "pd6"
  Bus Creator5/1 -> Bus Creator1/5  "pd5"
  Bus Creator4/1 -> Bus Creator1/4  "pd4"
  Bus Creator1/1 -> Fd2/1
  Constant6/1 -> Bus Creator3/1  "xx"
  Constant8/1 -> Bus Creator3/3  "xz"
  Constant7/1 -> Bus Creator3/2  "xy"
  Constant10/1 -> Bus Creator4/2  "xy"
  Constant11/1 -> Bus Creator4/3  "xz"
  Constant9/1 -> Bus Creator4/1  "xx"
  Constant14/1 -> Bus Creator5/1  "xx"
  Constant13/1 -> Bus Creator5/3  "xz"
  Constant12/1 -> Bus Creator5/2  "xy"
  Constant15/1 -> Bus Creator6/2  "xy"
  Constant16/1 -> Bus Creator6/3  "xz"
  Constant17/1 -> Bus Creator6/1  "xx"

== system chap05/Subsystem15/Subsystem14 ==
  note: % fx3 = [-2 0 0
      | % 2 0 0
      | % 3 0 0
      | % -3 0 0
      | % -1 0 0
      | % 1 0 0];
  Bus Creator{,2..6} (6 alike) : BusCreator  Inputs=3
  Bus Creator1 : BusCreator  Inputs=6
  Constant : Constant  Value=-2
  Constant{1..2,4..5,7..8,10..13,15..16} (12 alike) : Constant  Value=0
  Constant14 : Constant  Value=-1
  Constant17 : Constant
  Constant3 : Constant  Value=2
  Constant6 : Constant  Value=3
  Constant9 : Constant  Value=-3
  Fd3 : Outport
  wires:
  Constant/1 -> Bus Creator/1  "xx"
  Bus Creator/1 -> Bus Creator1/1  "pd1"
  Constant2/1 -> Bus Creator/3  "xz"
  Constant1/1 -> Bus Creator/2  "xy"
  Constant4/1 -> Bus Creator2/2  "xy"
  Constant5/1 -> Bus Creator2/3  "xz"
  Bus Creator2/1 -> Bus Creator1/2  "pd2"
  Constant3/1 -> Bus Creator2/1  "xx"
  Bus Creator3/1 -> Bus Creator1/3  "pd3"
  Bus Creator6/1 -> Bus Creator1/6  "pd6"
  Bus Creator5/1 -> Bus Creator1/5  "pd5"
  Bus Creator4/1 -> Bus Creator1/4  "pd4"
  Bus Creator1/1 -> Fd3/1
  Constant6/1 -> Bus Creator3/1  "xx"
  Constant8/1 -> Bus Creator3/3  "xz"
  Constant7/1 -> Bus Creator3/2  "xy"
  Constant10/1 -> Bus Creator4/2  "xy"
  Constant11/1 -> Bus Creator4/3  "xz"
  Constant9/1 -> Bus Creator4/1  "xx"
  Constant14/1 -> Bus Creator5/1  "xx"
  Constant13/1 -> Bus Creator5/3  "xz"
  Constant12/1 -> Bus Creator5/2  "xy"
  Constant15/1 -> Bus Creator6/2  "xy"
  Constant16/1 -> Bus Creator6/3  "xz"
  Constant17/1 -> Bus Creator6/1  "xx"

== system chap05/Subsystem15/Subsystem16 ==
  switch : Inport
  Add : Sum
  Constant1 : Constant  Value=0
  Data Store Memory : DataStoreMemory  ReadBeforeWriteMsg=warning  WriteAfterWriteMsg=warning  WriteAfterReadMsg=warning  ShowAdditionalParam=off
  Data Store Read : DataStoreRead  IndexOptions=Index vector (dialog)  Indices=1  OutputSizes=1
  Data Store Write : DataStoreWrite  IndexOptions=Index vector (dialog)  Indices=1  OutputSizes=1
  Switch : Switch  Criteria=u2 > Threshold
  t : Constant  Value=0.001
  time : Outport
  wires:
  Constant1/1 -> Switch/3
  Add/1 -> Data Store Write/1
  Switch/1 -> Add/1
  t/1 -> Switch/1
  switch/1 -> Switch/2
  Data Store Read/1 -> time/1, Add/2

== system chap05/Subsystem15/Subsystem8 ==
  note: % fx1 = [-1 1 0
      | % 0 1 0
      | % 1 1 0
      | % -1 -1 0
      | % 0 -1 0
      | % 1 -1 0];
  Bus Creator{,2..6} (6 alike) : BusCreator  Inputs=3
  Bus Creator1 : BusCreator  Inputs=6
  Constant{,9..10,12,15} (5 alike) : Constant  Value=-1
  Constant{1,4,6..7,17} (5 alike) : Constant
  Constant{2..3,5,8,11,13..14,16} (8 alike) : Constant  Value=0
  Fd1 : Outport
  wires:
  Constant17/1 -> Bus Creator6/1  "xx"
  Constant16/1 -> Bus Creator6/3  "xz"
  Constant15/1 -> Bus Creator6/2  "xy"
  Constant12/1 -> Bus Creator5/2  "xy"
  Constant13/1 -> Bus Creator5/3  "xz"
  Constant14/1 -> Bus Creator5/1  "xx"
  Constant9/1 -> Bus Creator4/1  "xx"
  Constant11/1 -> Bus Creator4/3  "xz"
  Constant10/1 -> Bus Creator4/2  "xy"
  Constant7/1 -> Bus Creator3/2  "xy"
  Constant8/1 -> Bus Creator3/3  "xz"
  Constant6/1 -> Bus Creator3/1  "xx"
  Bus Creator1/1 -> Fd1/1
  Bus Creator4/1 -> Bus Creator1/4  "pd4"
  Bus Creator5/1 -> Bus Creator1/5  "pd5"
  Bus Creator6/1 -> Bus Creator1/6  "pd6"
  Bus Creator3/1 -> Bus Creator1/3  "pd3"
  Constant3/1 -> Bus Creator2/1  "xx"
  Bus Creator2/1 -> Bus Creator1/2  "pd2"
  Constant5/1 -> Bus Creator2/3  "xz"
  Constant4/1 -> Bus Creator2/2  "xy"
  Constant1/1 -> Bus Creator/2  "xy"
  Constant2/1 -> Bus Creator/3  "xz"
  Bus Creator/1 -> Bus Creator1/1  "pd1"
  Constant/1 -> Bus Creator/1  "xx"

== system chap05/Subsystem16/Subsystem ==
  In19 : Inport
  switch : Inport  Port=2
  Bus Creator : BusCreator  Inputs=3
  Bus Selector : BusSelector  OutputSignals=state(tk).node1.xx,state(tk).node2.xx,state(tk).node3.xx,state(tk).node6.xx,state(tk).node1.vx,state(tk).node2.vx,state(tk).node3.vx,state(tk).node6.vx
  Bus Selector1 : BusSelector  OutputSignals=state(tk).node1.xy,state(tk).node2.xy,state(tk).node3.xy,state(tk).node6.xy,state(tk).node1.vy,state(tk).node2.vy,state(tk).node3.vy,state(tk).node6.vy
  Bus Selector2 : BusSelector  OutputSignals=state(tk).node1.xz,state(tk).node2.xz,state(tk).node3.xz,state(tk).node6.xz,state(tk).node1.vz,state(tk).node2.vz,state(tk).node3.vz,state(tk).node6.vz
  Bus Selector3 : BusSelector  OutputSignals=state(t).node1.vx
  Bus Selector4 : BusSelector  OutputSignals=state(t).node1.vy
  Bus Selector5 : BusSelector  OutputSignals=state(t).node1.vz
  Bus Selector6 : BusSelector  OutputSignals=state(t).node1.vx,state(t).node1.vy,state(t).node1.vz
  Bus Selector7 : BusSelector  OutputSignals=state(t).node1.vx,state(t).node1.vy,state(t).node1.vz
  Bus Selector8 : BusSelector  OutputSignals=control.node1.ux,control.node1.uy,control.node1.uz
  Subsystem1 : Subsystem
  Subsystem10 : Subsystem
  Subsystem11 : Subsystem
      settings: PortSchema="{\"entries\":[{\"content\":{\"sides\":[{\"content\":{\"connectorIds\":[\"In1\",\"In2\",\"In3\"]},\"type\":\"ConnectorPlacement.EquallySpacedRectSide\",\"uuid\":\"3c32f130-2df4-4697-80e9-267a8217898e\"},{\"content\":{\"connectorIds\":[\"Out1\"],\"side\":\"RIGHT\"},\"type\":\"ConnectorPlacement.EquallySpacedRectSide\",\"uuid\":\"840675a7-4714-440f-a6ce-75eff1b2763f\"},{\"content\":{\"connectorIds\":[\"In4\"],\"side\":\"TOP\"},\"type\":\"ConnectorPlacement.EquallySpacedRectSide\",\"uuid\":\"5c23af56-4ec3-4a39-a531-12998a0be3c8\"},{\"content\":{\"connectorIds\":[\"Out2\"],\"side\":\"BOTTOM\"},\"type\":\"ConnectorPlacement.EquallySpacedRectSide\",\"uuid\":\"31d953fb-65a0-42e9-a844-060de010f298\"}]},\"type\":\"ConnectorPlacement.EquallySpacedConnector\",\"uuid\":\"61b27aa3-5880-401e-bae3-4611093a191a\"}],\"packageUris\":[\"http://schema.mathworks.com/mf0/Connector/R2020b\"],\"version\":\"1.0\"}"
  Subsystem2 : Subsystem
  Subsystem3 : Subsystem
      settings: PortSchema="{\"entries\":[{\"content\":{\"sides\":[{\"content\":{\"connectorIds\":[\"In1\",\"In2\",\"In3\",\"In4\",\"In5\",\"In6\",\"In7\",\"In8\",\"In9\"]},\"type\":\"ConnectorPlacement.EquallySpacedRectSide\",\"uuid\":\"e02b19dc-feca-4a5f-b0a9-7b682689d3dc\"},{\"content\":{\"connectorIds\":[\"Out1\",\"Out2\",\"Out3\"],\"side\":\"RIGHT\"},\"type\":\"ConnectorPlacement.EquallySpacedRectSide\",\"uuid\":\"6cba16a1-1866-4332-a766-c6ecae75c00a\"},{\"content\":{\"connectorIds\":[],\"side\":\"TOP\"},\"type\":\"ConnectorPlacement.EquallySpacedRectSide\",\"uuid\":\"834934d8-ba7c-4cfc-8528-dda956d123e9\"},{\"content\":{\"connectorIds\":[\"In10\"],\"side\":\"BOTTOM\"},\"type\":\"ConnectorPlacement.EquallySpacedRectSide\",\"uuid\":\"a447ec2e-850c-49d1-98c5-4201d925b22c\"}]},\"type\":\"ConnectorPlacement.EquallySpacedConnector\",\"uuid\":\"dde62e81-0b86-43c6-8cdc-67ebf109c079\"}],\"packageUris\":[\"http://schema.mathworks.com/mf0/Connector/R2020b\"],\"version\":\"1.0\"}"
  Subsystem4 : Subsystem
      settings: PortSchema="{\"entries\":[{\"content\":{\"sides\":[{\"content\":{\"connectorIds\":[\"In1\",\"In2\",\"In3\"]},\"type\":\"ConnectorPlacement.EquallySpacedRectSide\",\"uuid\":\"3c32f130-2df4-4697-80e9-267a8217898e\"},{\"content\":{\"connectorIds\":[\"Out1\"],\"side\":\"RIGHT\"},\"type\":\"ConnectorPlacement.EquallySpacedRectSide\",\"uuid\":\"840675a7-4714-440f-a6ce-75eff1b2763f\"},{\"content\":{\"connectorIds\":[\"In4\"],\"side\":\"TOP\"},\"type\":\"ConnectorPlacement.EquallySpacedRectSide\",\"uuid\":\"5c23af56-4ec3-4a39-a531-12998a0be3c8\"},{\"content\":{\"connectorIds\":[\"Out2\"],\"side\":\"BOTTOM\"},\"type\":\"ConnectorPlacement.EquallySpacedRectSide\",\"uuid\":\"31d953fb-65a0-42e9-a844-060de010f298\"}]},\"type\":\"ConnectorPlacement.EquallySpacedConnector\",\"uuid\":\"61b27aa3-5880-401e-bae3-4611093a191a\"}],\"packageUris\":[\"http://schema.mathworks.com/mf0/Connector/R2020b\"],\"version\":\"1.0\"}"
  Subsystem6 : Subsystem
  Subsystem8 : Subsystem
      settings: PortSchema="{\"entries\":[{\"content\":{\"sides\":[{\"content\":{\"connectorIds\":[\"In1\",\"In2\",\"In3\",\"In4\",\"In5\",\"In6\"]},\"type\":\"ConnectorPlacement.EquallySpacedRectSide\",\"uuid\":\"6e2ae49e-f829-4a88-ba6d-12a1c984ff97\"},{\"content\":{\"connectorIds\":[\"Out1\"],\"side\":\"RIGHT\"},\"type\":\"ConnectorPlacement.EquallySpacedRectSide\",\"uuid\":\"1d02df48-94d5-4b75-9fdc-37bb62799324\"},{\"content\":{\"connectorIds\":[],\"side\":\"TOP\"},\"type\":\"ConnectorPlacement.EquallySpacedRectSide\",\"uuid\":\"e0c2a01b-94eb-432a-818f-b3ac4af71c3e\"},{\"content\":{\"connectorIds\":[\"In7\"],\"side\":\"BOTTOM\"},\"type\":\"ConnectorPlacement.EquallySpacedRectSide\",\"uuid\":\"1c8c54e5-1608-4962-a210-31f0a1951aa9\"}]},\"type\":\"ConnectorPlacement.EquallySpacedConnector\",\"uuid\":\"4e183442-7783-4f10-aa1a-c21f2f9b268a\"}],\"packageUris\":[\"http://schema.mathworks.com/mf0/Connector/R2020b\"],\"version\":\"1.0\"}"
  Subsystem9 : Subsystem
      settings: PortSchema="{\"entries\":[{\"content\":{\"sides\":[{\"content\":{\"connectorIds\":[\"In1\",\"In2\",\"In3\"]},\"type\":\"ConnectorPlacement.EquallySpacedRectSide\",\"uuid\":\"3c32f130-2df4-4697-80e9-267a8217898e\"},{\"content\":{\"connectorIds\":[\"Out1\"],\"side\":\"RIGHT\"},\"type\":\"ConnectorPlacement.EquallySpacedRectSide\",\"uuid\":\"840675a7-4714-440f-a6ce-75eff1b2763f\"},{\"content\":{\"connectorIds\":[\"In4\"],\"side\":\"TOP\"},\"type\":\"ConnectorPlacement.EquallySpacedRectSide\",\"uuid\":\"5c23af56-4ec3-4a39-a531-12998a0be3c8\"},{\"content\":{\"connectorIds\":[\"Out2\"],\"side\":\"BOTTOM\"},\"type\":\"ConnectorPlacement.EquallySpacedRectSide\",\"uuid\":\"31d953fb-65a0-42e9-a844-060de010f298\"}]},\"type\":\"ConnectorPlacement.EquallySpacedConnector\",\"uuid\":\"61b27aa3-5880-401e-bae3-4611093a191a\"}],\"packageUris\":[\"http://schema.mathworks.com/mf0/Connector/R2020b\"],\"version\":\"1.0\"}"
  u1 : Outport
  wires:
  Subsystem2/1(utx) -> Subsystem11/2(utz)
  Subsystem6/1(utx) -> Subsystem4/2(utx)
  Subsystem1/1(utx) -> Subsystem9/2(uty)
  Bus Creator/1 -> u1/1  "node1"
  In19/1 -> [state], Bus Selector2/1, Bus Selector/1, Bus Selector1/1
  Bus Selector/1 -> Subsystem6/1(xx1)  "<xx>"
  Bus Selector/2 -> Subsystem6/2(xx2)  "<xx>"
  Bus Selector/3 -> Subsystem6/3(xx3)  "<xx>"
  Bus Selector/4 -> Subsystem6/4(xx6)  "<xx>"
  Bus Selector/5 -> Subsystem6/5(vx1)  "<vx>"
  Bus Selector/6 -> Subsystem6/6(vx2)  "<vx>"
  Bus Selector/7 -> Subsystem6/7(vx3)  "<vx>"
  Bus Selector/8 -> Subsystem6/8(vx6)  "<vx>"
  Bus Selector1/1 -> Subsystem1/1(xy1)  "<xy>"
  Bus Selector1/2 -> Subsystem1/2(xy2)  "<xy>"
  Bus Selector1/3 -> Subsystem1/3(xy3)  "<xy>"
  Bus Selector1/4 -> Subsystem1/4(xy6)  "<xy>"
  Bus Selector1/5 -> Subsystem1/5(vy1)  "<vy>"
  Bus Selector1/6 -> Subsystem1/6(vy2)  "<vy>"
  Bus Selector1/7 -> Subsystem1/7(vy3)  "<vy>"
  Bus Selector1/8 -> Subsystem1/8(vy6)  "<vy>"
  Bus Selector2/1 -> Subsystem2/1(xz1)  "<xz>"
  Bus Selector2/2 -> Subsystem2/2(xx2)  "<xz>"
  Bus Selector2/3 -> Subsystem2/3(xz3)  "<xz>"
  Bus Selector2/4 -> Subsystem2/4(xz6)  "<xz>"
  Bus Selector2/5 -> Subsystem2/5(vz1)  "<vz>"
  Bus Selector2/6 -> Subsystem2/6(vz2)  "<vz>"
  Bus Selector2/7 -> Subsystem2/7(vz3)  "<vz>"
  Bus Selector2/8 -> Subsystem2/8(vz6)  "<vz>"
  [state] -> Bus Selector3/1
  Bus Selector3/1 -> Subsystem4/1(vx1)  "<vx>"
  Bus Selector4/1 -> Subsystem9/1(vy1)  "<vy>"
  [state] -> Bus Selector4/1
  [state] -> Bus Selector5/1
  Bus Selector5/1 -> Subsystem11/1(vz1)  "<vz>"
  [state] -> Bus Selector6/1
  Bus Selector6/2 -> Subsystem8/5(vy)  "<vy>"
  Bus Selector6/1 -> Subsystem8/4(vx)  "<vx>"
  Bus Selector6/3 -> Subsystem8/6(vz)  "<vz>"
  Subsystem8/1(" gain") -> [gain]  "p1"
  [gain] -> Subsystem11/3(gain)
  [gain] -> Subsystem9/3(gain)
  [gain] -> Subsystem4/3(gain)
  Subsystem4/2(Sx) -> [Sx]
  Subsystem9/2(Sz) -> [Sy]
  Subsystem11/2(Sz) -> [Sz]
  [Sx] -> Subsystem8/1(Sx)
  [Sy] -> Subsystem8/2(Sy)
  [Sz] -> Subsystem8/3(Sz)
  Subsystem10/1(ux) -> Bus Creator/1  "ux"
  Subsystem10/2(uy) -> Bus Creator/2  "uy"
  Subsystem10/3(uz) -> Bus Creator/3  "uz"
  Subsystem4/1(ux) -> Subsystem3/1(utx)
  Subsystem9/1(uy) -> Subsystem3/5(uty)
  Subsystem11/1(uz) -> Subsystem3/9(utz)
  [state] -> Bus Selector7/1
  Bus Selector7/1 -> Subsystem3/2(vx)  "<vx>"
  Bus Selector7/2 -> Subsystem3/3(vy)  "<vy>"
  Bus Selector7/3 -> Subsystem3/4(vz)  "<vz>"
  [state] -> Bus Selector8/1
  Bus Selector8/1 -> Subsystem3/6(ux)  "<ux>"
  Bus Selector8/2 -> Subsystem3/7(uy)  "<uy>"
  Bus Selector8/3 -> Subsystem3/8(uz)  "<uz>"
  Subsystem3/1(udtx) -> Subsystem10/1(utx)
  Subsystem3/2(udty) -> Subsystem10/2(uty)
  Subsystem3/3(udtz) -> Subsystem10/3(utz)
  switch/1 -> [switch], Subsystem4/4(switch)
  [switch] -> Subsystem9/4(switch)
  [switch] -> Subsystem11/4(switch)
  [switch] -> Subsystem3/10(switch)
  [switch] -> Subsystem8/7(switch)
